simulink model "a5TM3K52_A2"  (R2020b)
settings: Solver=VariableStepAuto  StartTime=0.0  StopTime=1  MaxStep=0.001  RelTol=1e-3
values from neighbouring files (symbols this model uses):
  c = 30000    [a5TM3A52_scr.m]
  h = 0.1    [a5TM3A52_scr.m]
  H = 0.3    [a5TM3A52_scr.m]
  m = 5    [a5TM3A52_scr.m]
undefined symbols (not defined in the file or in its folder): w0
settings Model: Creator=jakob  LastModifiedBy=jakob

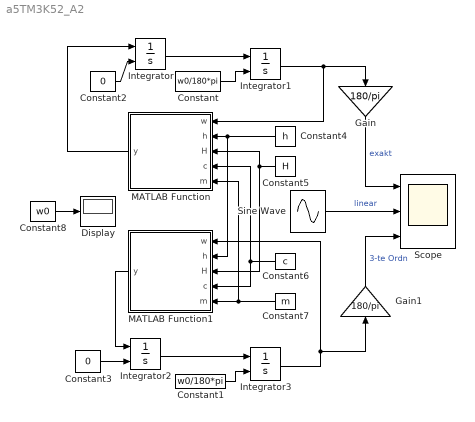
== system a5TM3K52_A2 ==
  Constant : Constant  Value=w0/180*pi
  Constant1 : Constant  Value=w0/180*pi
  Constant2 : Constant  Value=0
  Constant3 : Constant  Value=0
  Constant4 : Constant  Value=h
  Constant5 : Constant  Value=H
  Constant6 : Constant  Value=c
  Constant7 : Constant  Value=m
  Constant8 : Constant  Value=w0
  Display : Display
  Gain : Gain  Gain=180/pi
  Gain1 : Gain  Gain=180/pi
  Integrator{,1..3} (4 alike) : Integrator  InitialConditionSource=external
  MATLAB Function : MATLAB Function  TreatAsAtomicUnit=on
  MATLAB Function1 : MATLAB Function  TreatAsAtomicUnit=on
  Scope : Scope  NumInputPorts=3
  Sine Wave : Sin  Amplitude=w0  Frequency=sqrt((c*h^2-9.81*m*H)/(m*H^2))  Phase=pi/2  SampleTime=0
  wires:
  Integrator/1 -> Integrator1/1
  Integrator1/1 -> Gain/1, MATLAB Function/1(w)
  MATLAB Function/1(y) -> Integrator/1
  Integrator2/1 -> Integrator3/1
  Integrator3/1 -> MATLAB Function1/1(w), Gain1/1
  MATLAB Function1/1(y) -> Integrator2/1
  Constant/1 -> Integrator1/2
  Constant1/1 -> Integrator3/2
  Constant2/1 -> Integrator/2
  Constant3/1 -> Integrator2/2
  Constant4/1 -> MATLAB Function1/2(h), MATLAB Function/2(h)
  Constant5/1 -> MATLAB Function1/3(H), MATLAB Function/3(H)
  Constant6/1 -> MATLAB Function1/4(c), MATLAB Function/4(c)
  Constant7/1 -> MATLAB Function/5(m), MATLAB Function1/5(m)
  Gain/1 -> Scope/1  "exakt"
  Sine Wave/1 -> Scope/2  "linear"
  Gain1/1 -> Scope/3  "3-te Ordn"
  Constant8/1 -> Display/1

== matlab function a5TM3K52_A2/MATLAB Function1 ==
  data: w input; y output; h input; H input; c input; m input
function y = f_3_ordnung(w,h,H,c,m)

y = -(c*h^2-9.81*m*H)/(m*H^2)*w...
               +(4*c*h^2-9.81*m*H)/(6*m*H^2)*w^3;

== matlab function a5TM3K52_A2/MATLAB Function ==
  data: w input; y output; h input; H input; c input; m input
function y = fexact(w,h,H,c,m)
y = ( -c*h^2*sin(w)*cos(w) + m*H*9.81*sin(w) )/(m*H^2);
